simulink model "simple_vehicle_model"  (R2018b)
settings: Solver=VariableStepAuto  StartTime=0.0  StopTime=60  RelTol=1e-3
libraries: simulink x1
settings Model: Creator=Admin  LastModifiedBy=Admin

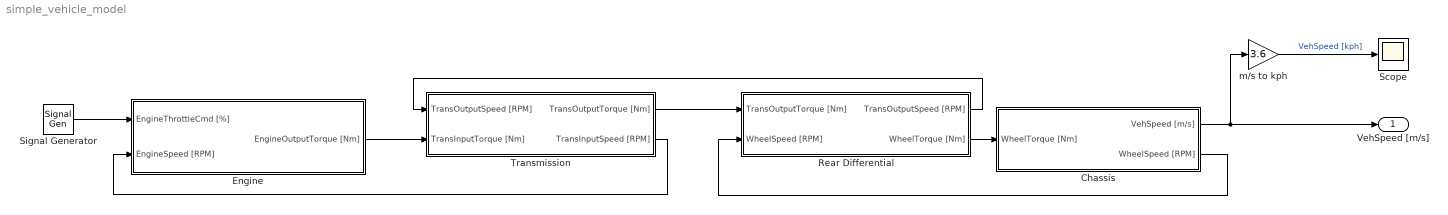
== system simple_vehicle_model ==
  Chassis : Subsystem
  Engine : Subsystem
  Rear Differential : Subsystem
  Scope : Scope
  Signal Generator : SignalGenerator  WaveForm=square  Amplitude=50  Frequency=0.1
  Transmission : Subsystem
  m/s to kph : Gain  Gain=3.6
  VehSpeed [m/s] : Outport
  wires:
  Rear Differential/2(WheelTorque [Nm]) -> Chassis/1(WheelTorque [Nm])
  Chassis/1(VehSpeed [m/s]) -> VehSpeed [m/s]/1, m/s to kph/1
  Transmission/1(TransOutputTorque [Nm]) -> Rear Differential/1(TransOutputTorque [Nm])
  Chassis/2(WheelSpeed [RPM]) -> Rear Differential/2(WheelSpeed [RPM])
  Rear Differential/1(TransOutputSpeed [RPM]) -> Transmission/1(TransOutputSpeed [RPM])
  Engine/1(EngineOutputTorque [Nm]) -> Transmission/2(TransInputTorque [Nm])
  Transmission/2(TransInputSpeed [RPM]) -> Engine/2(EngineSpeed [RPM])
  Signal Generator/1 -> Engine/1(EngineThrottleCmd [%])
  m/s to kph/1 -> Scope/1  "VehSpeed [kph]"

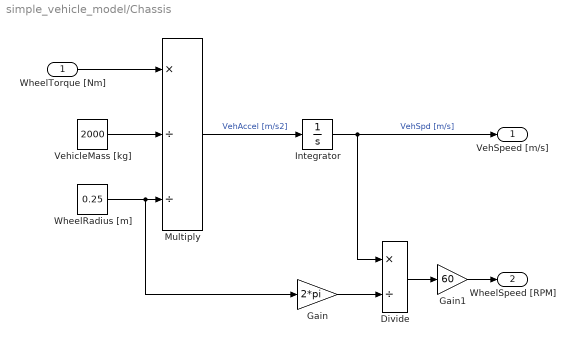
== system simple_vehicle_model/Chassis ==
  WheelTorque [Nm] : Inport
  Divide : Product  Inputs=*/
  Gain : Gain  Gain=2*pi
  Gain1 : Gain  Gain=60
  Integrator : Integrator
  Multiply : Product  Inputs=*//
  VehicleMass [kg] : Constant  Value=2000
  WheelRadius [m] : Constant  Value=0.25
  VehSpeed [m/s] : Outport
  WheelSpeed [RPM] : Outport  Port=2
  wires:
  Multiply/1 -> Integrator/1  "VehAccel [m/s2]"
  VehicleMass [kg]/1 -> Multiply/2
  WheelTorque [Nm]/1 -> Multiply/1
  WheelRadius [m]/1 -> Gain/1, Multiply/3
  Integrator/1 -> Divide/1, VehSpeed [m/s]/1  "VehSpd [m/s]"
  Gain/1 -> Divide/2
  Divide/1 -> Gain1/1
  Gain1/1 -> WheelSpeed [RPM]/1

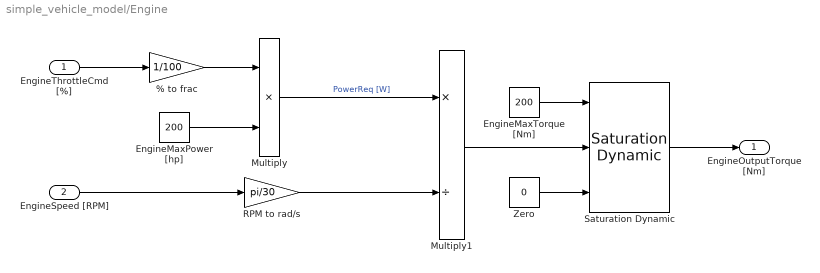
== system simple_vehicle_model/Engine ==
  EngineThrottleCmd [%] : Inport
  EngineSpeed [RPM] : Inport  Port=2
  % to frac : Gain  Gain=1/100
  EngineMaxPower [hp] : Constant  Value=200
  EngineMaxTorque [Nm] : Constant  Value=200
  Multiply : Product
  Multiply1 : Product  Inputs=*/
  RPM to rad/s : Gain  Gain=pi/30
  Saturation Dynamic : simulink/Discontinuities/Saturation Dynamic  OutMin=[]  OutMax=[]  OutDataTypeStr=Inherit: Same as second input  OutDataType=fixdt(1, 16)  OutScaling=2^-10  DoSatur=off
  Zero : Constant  Value=0
  EngineOutputTorque [Nm] : Outport
  wires:
  RPM to rad/s/1 -> Multiply1/2
  EngineSpeed [RPM]/1 -> RPM to rad/s/1
  EngineMaxPower [hp]/1 -> Multiply/2
  % to frac/1 -> Multiply/1
  EngineThrottleCmd [%]/1 -> % to frac/1
  Multiply/1 -> Multiply1/1  "PowerReq [W]"
  Multiply1/1 -> Saturation Dynamic/2
  Saturation Dynamic/1 -> EngineOutputTorque [Nm]/1
  EngineMaxTorque [Nm]/1 -> Saturation Dynamic/1
  Zero/1 -> Saturation Dynamic/3

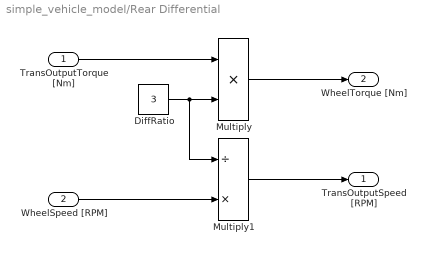
== system simple_vehicle_model/Rear Differential ==
  TransOutputTorque [Nm] : Inport
  WheelSpeed [RPM] : Inport  Port=2
  DiffRatio : Constant  Value=3
  Multiply : Product
  Multiply1 : Product  Inputs=/*
  TransOutputSpeed [RPM] : Outport
  WheelTorque [Nm] : Outport  Port=2
  wires:
  DiffRatio/1 -> Multiply1/1, Multiply/2
  TransOutputTorque [Nm]/1 -> Multiply/1
  Multiply/1 -> WheelTorque [Nm]/1
  WheelSpeed [RPM]/1 -> Multiply1/2
  Multiply1/1 -> TransOutputSpeed [RPM]/1

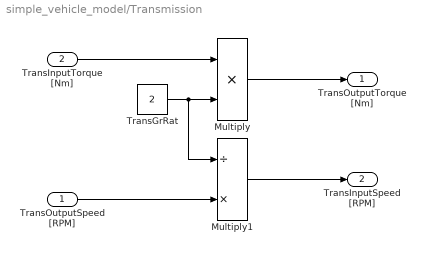
== system simple_vehicle_model/Transmission ==
  TransOutputSpeed [RPM] : Inport
  TransInputTorque [Nm] : Inport  Port=2
  Multiply : Product
  Multiply1 : Product  Inputs=/*
  TransGrRat : Constant  Value=2
  TransOutputTorque [Nm] : Outport
  TransInputSpeed [RPM] : Outport  Port=2
  wires:
  Multiply1/1 -> TransInputSpeed [RPM]/1
  TransOutputSpeed [RPM]/1 -> Multiply1/2
  Multiply/1 -> TransOutputTorque [Nm]/1
  TransInputTorque [Nm]/1 -> Multiply/1
  TransGrRat/1 -> Multiply/2, Multiply1/1
